simulink model "gm_DSM_MOD8_HDL"  (R2013b)
settings: Solver=FixedStepDiscrete  SolverMode=SingleTasking  StartTime=0.0  StopTime=N/Fs  RelTol=1e-3
undefined symbols (not defined in the file or in its folder): a, b, c, g
settings Model: Creator=o_cotte  LastModifiedBy=o_cotte
settings OptimizationCC: BlockReduction=off  BooleanDataType=off  ConditionallyExecuteInputs=off
settings DebuggingCC: SaveWithParameterizedLinksMsg=none  SignalResolutionControl=TryResolveAllWithWarning  SolverPrmCheckMsg=none  MultiTaskDSMMsg=warning  MultiTaskCondExecSysMsg=none
settings HardwareCC: TargetUnknown=on
settings RTWCC: IncludeERTFirstTime=on

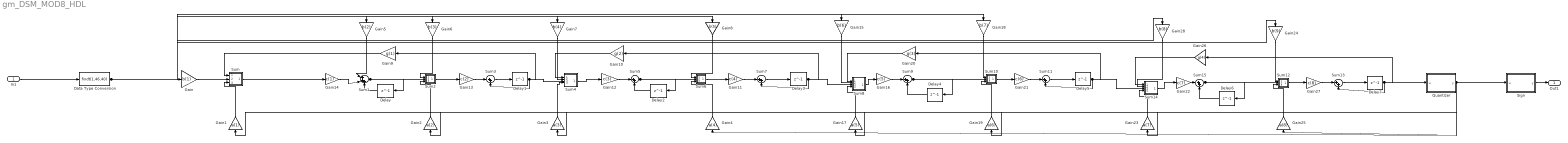
== system gm_DSM_MOD8_HDL ==
  In1 : Inport
  Data Type Conversion : DataTypeConversion  OutDataTypeStr=fixdt(1,46,40)
  Delay{,1..7} (8 alike) : Delay  DelayLength=1  InitialCondition=0
  Gain : Gain  Gain=b(1)  OutDataTypeStr=Inherit: Same as input  ParamDataTypeStr=Inherit: Same as input  LockScale=on
  Gain1 : Gain  Gain=a(1)  OutDataTypeStr=Inherit: Same as input
  Gain10 : Gain  Gain=g(2)  OutDataTypeStr=Inherit: Same as input  ParamDataTypeStr=Inherit: Same as input  LockScale=on
  Gain11 : Gain  Gain=c(4)  OutDataTypeStr=Inherit: Same as input  ParamDataTypeStr=Inherit: Same as input  LockScale=on
  Gain12 : Gain  Gain=c(3)  OutDataTypeStr=Inherit: Same as input  ParamDataTypeStr=Inherit: Same as input  LockScale=on
  Gain13 : Gain  Gain=c(2)  OutDataTypeStr=Inherit: Same as input  ParamDataTypeStr=Inherit: Same as input  LockScale=on
  Gain14 : Gain  Gain=c(1)  OutDataTypeStr=Inherit: Same as input  ParamDataTypeStr=Inherit: Same as input  LockScale=on
  Gain15 : Gain  Gain=b(6)  OutDataTypeStr=Inherit: Same as input  ParamDataTypeStr=Inherit: Same as input  LockScale=on
  Gain16 : Gain  Gain=c(5)  OutDataTypeStr=Inherit: Same as input  ParamDataTypeStr=Inherit: Same as input  LockScale=on
  Gain17 : Gain  Gain=a(5)  OutDataTypeStr=Inherit: Same as input
  Gain18 : Gain  Gain=b(7)  OutDataTypeStr=Inherit: Same as input  ParamDataTypeStr=Inherit: Same as input  LockScale=on
  Gain19 : Gain  Gain=a(6)  OutDataTypeStr=Inherit: Same as input
  Gain2 : Gain  Gain=a(2)  OutDataTypeStr=Inherit: Same as input
  Gain20 : Gain  Gain=g(3)  OutDataTypeStr=Inherit: Same as input  ParamDataTypeStr=Inherit: Same as input  LockScale=on
  Gain21 : Gain  Gain=c(6)  OutDataTypeStr=Inherit: Same as input  ParamDataTypeStr=Inherit: Same as input  LockScale=on
  Gain22 : Gain  Gain=c(7)  OutDataTypeStr=Inherit: Same as input  ParamDataTypeStr=Inherit: Same as input  LockScale=on
  Gain23 : Gain  Gain=a(7)  OutDataTypeStr=Inherit: Same as input
  Gain24 : Gain  Gain=b(9)  OutDataTypeStr=Inherit: Same as input  ParamDataTypeStr=Inherit: Same as input  LockScale=on
  Gain25 : Gain  Gain=a(8)  OutDataTypeStr=Inherit: Same as input
  Gain26 : Gain  Gain=g(4)  OutDataTypeStr=Inherit: Same as input  ParamDataTypeStr=Inherit: Same as input  LockScale=on
  Gain27 : Gain  Gain=c(8)  OutDataTypeStr=Inherit: Same as input  ParamDataTypeStr=Inherit: Same as input  LockScale=on
  Gain28 : Gain  Gain=b(8)  OutDataTypeStr=Inherit: Same as input  ParamDataTypeStr=Inherit: Same as input  LockScale=on
  Gain3 : Gain  Gain=a(3)  OutDataTypeStr=Inherit: Same as input
  Gain4 : Gain  Gain=a(4)  OutDataTypeStr=Inherit: Same as input
  Gain5 : Gain  Gain=b(2)  OutDataTypeStr=Inherit: Same as input  ParamDataTypeStr=Inherit: Same as input  LockScale=on
  Gain6 : Gain  Gain=b(3)  OutDataTypeStr=Inherit: Same as input  ParamDataTypeStr=Inherit: Same as input  LockScale=on
  Gain7 : Gain  Gain=b(4)  OutDataTypeStr=Inherit: Same as input  ParamDataTypeStr=Inherit: Same as input  LockScale=on
  Gain8 : Gain  Gain=b(5)  OutDataTypeStr=Inherit: Same as input  ParamDataTypeStr=Inherit: Same as input  LockScale=on
  Gain9 : Gain  Gain=g(1)  OutDataTypeStr=Inherit: Same as input  ParamDataTypeStr=Inherit: Same as input  LockScale=on
  Quantizer : Subsystem
  Sign : Subsystem
  Sum : Subsystem
  Sum1 : Sum  Inputs=|+++  OutDataTypeStr=Inherit: Same as accumulator  LockScale=on
  Sum10 : Subsystem
  Sum{3,5,7,9,11,13,15} (7 alike) : Sum  Inputs=|++  OutDataTypeStr=Inherit: Same as accumulator  LockScale=on
  Sum12 : Subsystem
  Sum14 : Subsystem
  Sum2 : Subsystem
  Sum4 : Subsystem
  Sum6 : Subsystem
  Sum8 : Subsystem
  Out1 : Outport
  wires:
  In1/1 -> Data Type Conversion/1
  Data Type Conversion/1 -> Gain8/1, Gain7/1, Gain6/1, Gain5/1, Gain28/1, Gain24/1, Gain18/1, Gain15/1, Gain/1
  Delay/1 -> Sum1/3
  Delay1/1 -> Sum4/3(In3), Sum3/2, Gain9/1
  Delay2/1 -> Sum5/2
  Delay3/1 -> Sum8/3(In3), Sum7/2, Gain10/1
  Delay4/1 -> Sum9/2
  Delay5/1 -> Sum14/3(In3), Sum11/2, Gain20/1
  Delay6/1 -> Sum15/2
  Delay7/1 -> Sum13/2, Gain26/1, Quantizer/1(u)
  Gain/1 -> Sum/2(In2)
  Gain1/1 -> Sum/3(In3)
  Gain10/1 -> Sum4/1(In1)
  Gain11/1 -> Sum7/1
  Gain12/1 -> Sum5/1
  Gain13/1 -> Sum3/1
  Gain14/1 -> Sum1/2
  Gain15/1 -> Sum8/2(In2)
  Gain16/1 -> Sum9/1
  Gain17/1 -> Sum8/4(In4)
  Gain18/1 -> Sum10/1(In1)
  Gain19/1 -> Sum10/3(In3)
  Gain2/1 -> Sum2/3(In3)
  Gain20/1 -> Sum8/1(In1)
  Gain21/1 -> Sum11/1
  Gain22/1 -> Sum15/1
  Gain23/1 -> Sum14/4(In4)
  Gain24/1 -> Sum12/1(In1)
  Gain25/1 -> Sum12/3(In3)
  Gain26/1 -> Sum14/1(In1)
  Gain27/1 -> Sum13/1
  Gain28/1 -> Sum14/2(In2)
  Gain3/1 -> Sum4/4(In4)
  Gain4/1 -> Sum6/3(In3)
  Gain5/1 -> Sum1/1
  Gain6/1 -> Sum2/1(In1)
  Gain7/1 -> Sum4/2(In2)
  Gain8/1 -> Sum6/1(In1)
  Gain9/1 -> Sum/1(In1)
  Quantizer/1(y) -> Gain4/1, Gain3/1, Gain25/1, Gain23/1, Gain2/1, Gain19/1, Gain17/1, Gain1/1, Sign/1(u)
  Sign/1(y) -> Out1/1
  Sum/1(Out1) -> Gain14/1
  Sum1/1 -> Sum2/2(In2), Delay/1
  Sum10/1(Out1) -> Gain21/1
  Sum11/1 -> Delay5/1
  Sum12/1(Out1) -> Gain27/1
  Sum13/1 -> Delay7/1
  Sum14/1(Out1) -> Gain22/1
  Sum15/1 -> Sum12/2(In2), Delay6/1
  Sum2/1(Out1) -> Gain13/1
  Sum3/1 -> Delay1/1
  Sum4/1(Out1) -> Gain12/1
  Sum5/1 -> Sum6/2(In2), Delay2/1
  Sum6/1(Out1) -> Gain11/1
  Sum7/1 -> Delay3/1
  Sum8/1(Out1) -> Gain16/1
  Sum9/1 -> Sum10/2(In2), Delay4/1

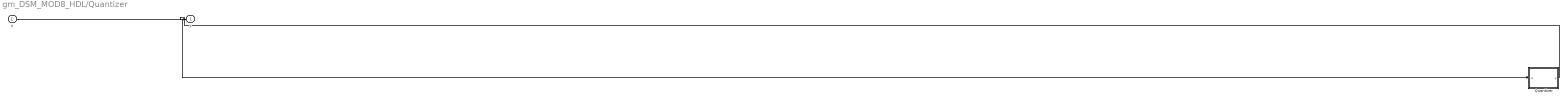
== system gm_DSM_MOD8_HDL/Quantizer ==
  u : Inport
  Quantizer : MATLAB Function  TreatAsAtomicUnit=on
  y : Outport
  wires:
  u/1 -> Quantizer/1(u)
  Quantizer/1(y) -> y/1

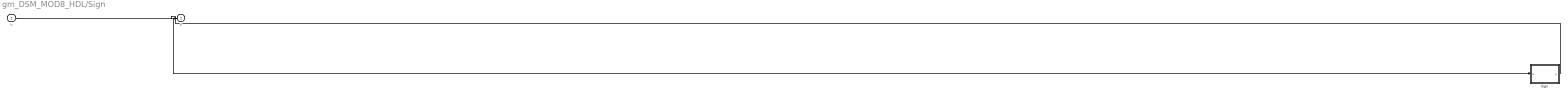
== system gm_DSM_MOD8_HDL/Sign ==
  u : Inport
  Sign : MATLAB Function  TreatAsAtomicUnit=on
  y : Outport
  wires:
  u/1 -> Sign/1(u)
  Sign/1(y) -> y/1

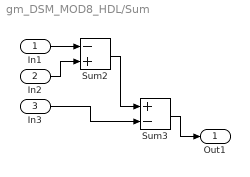
== system gm_DSM_MOD8_HDL/Sum ==
  In1 : Inport  OutDataTypeStr=fixdt('sfix46_En40')
  In2 : Inport  Port=2  OutDataTypeStr=fixdt('sfix46_En40')
  In3 : Inport  Port=3  OutDataTypeStr=fixdt('sfix46_En40')
  Sum2 : Sum  Inputs=-+  AccumDataTypeStr=fixdt(1,46,40)  OutDataTypeStr=fixdt(1,46,40)
  Sum3 : Sum  Inputs=+-  AccumDataTypeStr=fixdt(1,46,40)  OutDataTypeStr=fixdt(1,46,40)
  Out1 : Outport
  wires:
  In1/1 -> Sum2/1
  In2/1 -> Sum2/2
  Sum2/1 -> Sum3/1
  In3/1 -> Sum3/2
  Sum3/1 -> Out1/1

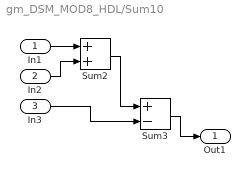
== system gm_DSM_MOD8_HDL/Sum10 ==
  In1 : Inport  OutDataTypeStr=fixdt('sfix46_En40')
  In2 : Inport  Port=2  OutDataTypeStr=fixdt('sfix46_En40')
  In3 : Inport  Port=3  OutDataTypeStr=fixdt('sfix46_En40')
  Sum2 : Sum  AccumDataTypeStr=fixdt(1,46,40)  OutDataTypeStr=fixdt(1,46,40)
  Sum3 : Sum  Inputs=+-  AccumDataTypeStr=fixdt(1,46,40)  OutDataTypeStr=fixdt(1,46,40)
  Out1 : Outport
  wires:
  In1/1 -> Sum2/1
  In2/1 -> Sum2/2
  Sum2/1 -> Sum3/1
  In3/1 -> Sum3/2
  Sum3/1 -> Out1/1

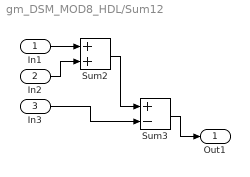
== system gm_DSM_MOD8_HDL/Sum12 ==
  In1 : Inport  OutDataTypeStr=fixdt('sfix46_En40')
  In2 : Inport  Port=2  OutDataTypeStr=fixdt('sfix46_En40')
  In3 : Inport  Port=3  OutDataTypeStr=fixdt('sfix46_En40')
  Sum2 : Sum  AccumDataTypeStr=fixdt(1,46,40)  OutDataTypeStr=fixdt(1,46,40)
  Sum3 : Sum  Inputs=+-  AccumDataTypeStr=fixdt(1,46,40)  OutDataTypeStr=fixdt(1,46,40)
  Out1 : Outport
  wires:
  In1/1 -> Sum2/1
  In2/1 -> Sum2/2
  Sum2/1 -> Sum3/1
  In3/1 -> Sum3/2
  Sum3/1 -> Out1/1

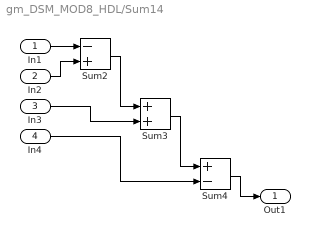
== system gm_DSM_MOD8_HDL/Sum14 ==
  In1 : Inport  OutDataTypeStr=fixdt('sfix46_En40')
  In2 : Inport  Port=2  OutDataTypeStr=fixdt('sfix46_En40')
  In3 : Inport  Port=3  OutDataTypeStr=fixdt('sfix46_En40')
  In4 : Inport  Port=4  OutDataTypeStr=fixdt('sfix46_En40')
  Sum2 : Sum  Inputs=-+  AccumDataTypeStr=fixdt(1,46,40)  OutDataTypeStr=fixdt(1,46,40)
  Sum3 : Sum  AccumDataTypeStr=fixdt(1,46,40)  OutDataTypeStr=fixdt(1,46,40)
  Sum4 : Sum  Inputs=+-  AccumDataTypeStr=fixdt(1,46,40)  OutDataTypeStr=fixdt(1,46,40)
  Out1 : Outport
  wires:
  In1/1 -> Sum2/1
  In2/1 -> Sum2/2
  Sum2/1 -> Sum3/1
  In3/1 -> Sum3/2
  Sum3/1 -> Sum4/1
  In4/1 -> Sum4/2
  Sum4/1 -> Out1/1

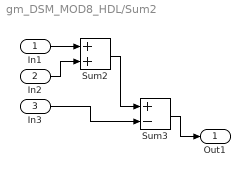
== system gm_DSM_MOD8_HDL/Sum2 ==
  In1 : Inport  OutDataTypeStr=fixdt('sfix46_En40')
  In2 : Inport  Port=2  OutDataTypeStr=fixdt('sfix46_En40')
  In3 : Inport  Port=3  OutDataTypeStr=fixdt('sfix46_En40')
  Sum2 : Sum  AccumDataTypeStr=fixdt(1,46,40)  OutDataTypeStr=fixdt(1,46,40)
  Sum3 : Sum  Inputs=+-  AccumDataTypeStr=fixdt(1,46,40)  OutDataTypeStr=fixdt(1,46,40)
  Out1 : Outport
  wires:
  In1/1 -> Sum2/1
  In2/1 -> Sum2/2
  Sum2/1 -> Sum3/1
  In3/1 -> Sum3/2
  Sum3/1 -> Out1/1

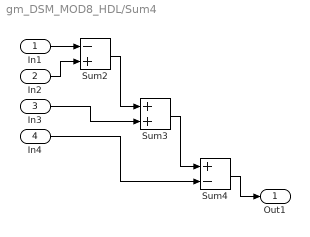
== system gm_DSM_MOD8_HDL/Sum4 ==
  In1 : Inport  OutDataTypeStr=fixdt('sfix46_En40')
  In2 : Inport  Port=2  OutDataTypeStr=fixdt('sfix46_En40')
  In3 : Inport  Port=3  OutDataTypeStr=fixdt('sfix46_En40')
  In4 : Inport  Port=4  OutDataTypeStr=fixdt('sfix46_En40')
  Sum2 : Sum  Inputs=-+  AccumDataTypeStr=fixdt(1,46,40)  OutDataTypeStr=fixdt(1,46,40)
  Sum3 : Sum  AccumDataTypeStr=fixdt(1,46,40)  OutDataTypeStr=fixdt(1,46,40)
  Sum4 : Sum  Inputs=+-  AccumDataTypeStr=fixdt(1,46,40)  OutDataTypeStr=fixdt(1,46,40)
  Out1 : Outport
  wires:
  In1/1 -> Sum2/1
  In2/1 -> Sum2/2
  Sum2/1 -> Sum3/1
  In3/1 -> Sum3/2
  Sum3/1 -> Sum4/1
  In4/1 -> Sum4/2
  Sum4/1 -> Out1/1

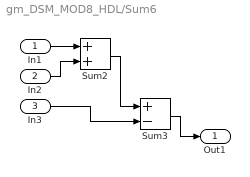
== system gm_DSM_MOD8_HDL/Sum6 ==
  In1 : Inport  OutDataTypeStr=fixdt('sfix46_En40')
  In2 : Inport  Port=2  OutDataTypeStr=fixdt('sfix46_En40')
  In3 : Inport  Port=3  OutDataTypeStr=fixdt('sfix46_En40')
  Sum2 : Sum  AccumDataTypeStr=fixdt(1,46,40)  OutDataTypeStr=fixdt(1,46,40)
  Sum3 : Sum  Inputs=+-  AccumDataTypeStr=fixdt(1,46,40)  OutDataTypeStr=fixdt(1,46,40)
  Out1 : Outport
  wires:
  In1/1 -> Sum2/1
  In2/1 -> Sum2/2
  Sum2/1 -> Sum3/1
  In3/1 -> Sum3/2
  Sum3/1 -> Out1/1

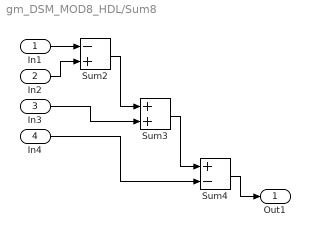
== system gm_DSM_MOD8_HDL/Sum8 ==
  In1 : Inport  OutDataTypeStr=fixdt('sfix46_En40')
  In2 : Inport  Port=2  OutDataTypeStr=fixdt('sfix46_En40')
  In3 : Inport  Port=3  OutDataTypeStr=fixdt('sfix46_En40')
  In4 : Inport  Port=4  OutDataTypeStr=fixdt('sfix46_En40')
  Sum2 : Sum  Inputs=-+  AccumDataTypeStr=fixdt(1,46,40)  OutDataTypeStr=fixdt(1,46,40)
  Sum3 : Sum  AccumDataTypeStr=fixdt(1,46,40)  OutDataTypeStr=fixdt(1,46,40)
  Sum4 : Sum  Inputs=+-  AccumDataTypeStr=fixdt(1,46,40)  OutDataTypeStr=fixdt(1,46,40)
  Out1 : Outport
  wires:
  In1/1 -> Sum2/1
  In2/1 -> Sum2/2
  Sum2/1 -> Sum3/1
  In3/1 -> Sum3/2
  Sum3/1 -> Sum4/1
  In4/1 -> Sum4/2
  Sum4/1 -> Out1/1

== matlab function gm_DSM_MOD8_HDL/Sign/Sign ==
  data: u input; y output
function y = fcn(u)
%#codegen
if u < 0
    y = fi(-1,1,2,0);
else
    y = fi(1,1,2,0);
end

== matlab function gm_DSM_MOD8_HDL/Quantizer/Quantizer ==
  data: u input; y output
function y = fcn(u)
%#codegen
if u < 0
    y = fi(-1,1,46,40);
else
    y = fi(1,1,46,40);
end
